simulink model "phase4_scheduler_testbed"  (R2026a)
settings: Solver=VariableStepAuto  StopTime=0.1  SampleTimeConstraint=Specified  EnableMultiTasking=on
undefined symbols (not defined in the file): D1, D3, initialControllerMeasurement, m, n, P, SupervisorTask
libraries: proctasklib x1
settings Model: Creator=The MathWorks, Inc.  LastModifiedBy=rayyu
settings SolverCC: PositivePriorityOrder=on
settings DebuggingCC: SignalInfNanChecking=error
settings HardwareCC: ProdBitPerLong=64.0  ProdLargestAtomicInteger=LongLong  ProdLargestAtomicFloat=Double  ProdHWDeviceType=ARM Compatible->ARM Cortex-A (64-bit)  HardwareBoardFeatureSet=SoCBlockset
settings RTWCC: SystemTargetFile=ert.tlc  HardwareBoard=Xilinx Zynq UltraScale+ MPSoC ZCU102 Evaluation Kit  TLCOptions="-aInlineSetEventsForThisBaseRateFcn=TLC_FALSE -aSuppressMultiTaskScheduler=TLC_FALSE  -aRateBasedStepFcn=0"  GenerateReport=on  Toolchain=Linaro AArch64 Linux v6.3.1  IncludeHyperlinkInReport=on  LaunchReport=on  GenerateTraceInfo=on  GenerateTraceReport=on  GenerateTraceReportSl=on  GenerateTraceReportSf=on  GenerateTraceReportEml=on  Description=Embedded Coder
settings ERTTargetCC: ExtModeTransport=2.0  DynamicArrayContainerType=coder::array

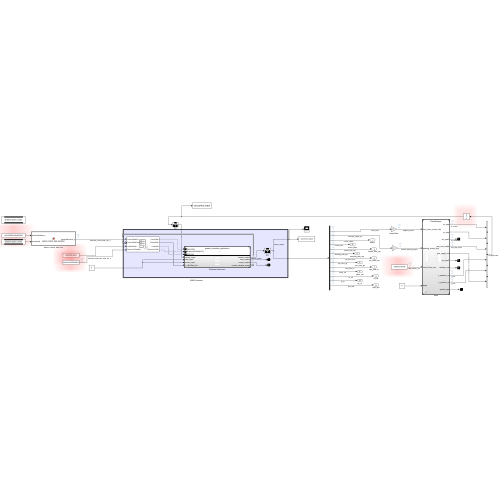
[thumbnail: Simulink's stored preview of the top-level diagram]
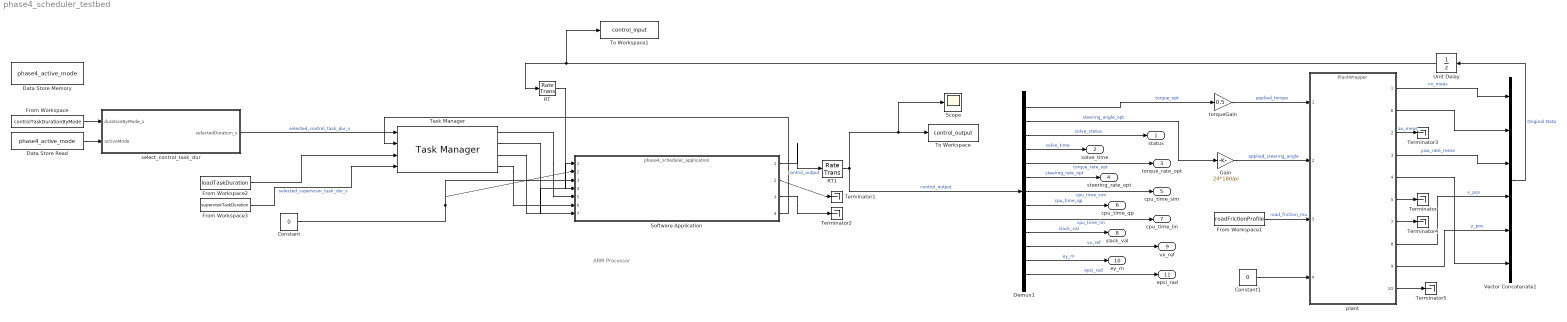
== system phase4_scheduler_testbed ==
  note: ARM Processor
  Constant : Constant  Value=0
  Constant1 : Constant  Value=0
  Data Store Memory : DataStoreMemory  DataStoreName=phase4_active_mode  WriteAfterWriteMsg=warning  InitialValue=3  ShowAdditionalParam=off  OutDataTypeStr=uint8  Dimensions=1
  Data Store Read : DataStoreRead  DataStoreName=phase4_active_mode  IndexOptions=Index vector (dialog)  Indices=1  OutputSizes=1
  Demux1 : Demux  Outputs=[1 1 1 1 1 1 1 1 1 4 1 1 1]
  From Workspace : FromWorkspace  VariableName=controlTaskDurationByMode  Interpolate=off  OutputAfterFinalValue=Holding final value
  From Workspace1 : FromWorkspace  VariableName=roadFrictionProfile  SampleTime=0.01  Interpolate=off  OutputAfterFinalValue=Holding final value
  From Workspace2 : FromWorkspace  VariableName=loadTaskDuration  Interpolate=off  OutputAfterFinalValue=Holding final value
  From Workspace3 : FromWorkspace  VariableName=supervisorTaskDuration  Interpolate=off  OutputAfterFinalValue=Holding final value
  Gain : Gain  Gain=24*180/pi
  RT : RateTransition  Deterministic=off
  RT1 : RateTransition  Deterministic=off
  Scope : Scope
      settings: ActiveDisplayYMinimum=-2.25  ActiveDisplayYMaximum=0.24999999999999994
  Software Application : ModelReference  OutputPortMessageModes=n,n,n,m  ModelNameDialog=phase4_scheduler_application.slx  SimulationMode=Normal  ScheduleRates=on  CachedPortDiscreteRates={'',0.005;'SupervisorTask',0.01;'',0.05}  ModelEventPortInfo=P:D1[0.005][0][0],P:SupervisorTask[0.01][1][0],P:D3[0.05][0][0]  HasExplicitPartitions=on  ModelReferenceVersion=14.163
  Task Manager : proctasklib/Task Manager  AllTaskData="[{\"taskName\":\"CommTask\",\"taskType\":\"Timer-driven\",\"taskEvent\":\"CommTaskEvent\",\"taskPeriod\":\"0.005\",\"taskPriority\":\"50\",\"coreSelection\":\"Specified core\",\"coreNum\":\"0\",\"dropOverranTasks\":false,\"playbackRecorded\":false,\"diagnosticsFile\":\"\",\"taskDurationSource\":\"Dialog\",\"taskDuration\":1E-6,\"taskDurationDeviation\":0,\"logExecutionData\":true,\"logDroppedTasks\":false,\"version\":\"2.6\",\"taskDurationData\":{\"percent\":\"100\",\"mean\":\"0.0005\",\"dev\":\"0\",\"min\":\"0.0005\",\"max\":\"0.0005\"},\"taskEventSource\":\"Internal\",\"taskEventSourceAssignmentType\":\"AutoAssigned\",\"taskEventSourceType\":\"Unspecified\",\"taskEventGroup\":\"Unspecified\",\"taskEventInterrupt\":\"Unspecified\",\"taskEventOrder\":1,\"taskDisablePremption\":false,\"taskClearInterruptFlagsAtEndOfEvent\":false},{\"taskName\":\"ControlTask\",\"taskType\":\"Event-driven\",\"taskEvent\":\"ControlTaskEvent\",\"taskPeriod\":\"0.01\",\"taskPriority\":\"50\",\"coreSelection\":\"Specified core\",\"coreNum\":\"0\",\"dropOverranTasks\":false,\"playbackRecorded\":false,\"diagnosticsFile\":\"\",\"taskDurationSource\":\"Input port\",\"taskDuration\":1E-6,\"taskDurationDeviation\":0,\"logExecutionData\":true,\"logDroppedTasks\":false,\"version\":\"2.6\",\"taskDurationData\":{\"percent\":\"100\",\"mean\":\"1e-06\",\"dev\":\"0\",\"min\":\"1e-06\",\"max\":\"1e-06\"},\"taskEventSource\":\"Unspecified\",\"taskEventSourceAssignmentType\":\"Unassigned\",\"taskEventSourceType\":\"Unspecified\",\"taskEventGroup\":\"Unspecified\",\"taskEventInterrupt\":\"Unspecified\",\"taskEventOrder\":1,\"taskDisablePremption\":false,\"taskClearInterruptFlagsAtEndOfEvent\":false},{\"taskName\":\"LoadTask\",\"taskType\":\"Timer-driven\",\"taskEvent\":\"newTask1Event\",\"taskPeriod\":\"0.05\",\"taskPriority\":\"50\",\"coreSelection\":\"Specified core\",\"coreNum\":\"0\",\"dropOverranTasks\":false,\"playbackRecorded\":false,\"diagnosticsFile\":\"\",\"taskDurationSource\":\"Input port\",\"taskDuration\":1E-6,\"taskDurationDeviation\":0,\"logExecutionData\":true,\"logDroppedTasks\":false,\"version\":\"2.6\",\"taskDurationData\":{\"percent\":\"100\",\"mean\":\"1e-06\",\"dev\":\"0\",\"min\":\"1e-06\",\"max\":\"1e-06\"},\"taskEventSource\":\"Internal\",\"taskEventSourceAssignmentType\":\"AutoAssigned\",\"taskEventSourceType\":\"Unspecified\",\"taskEventGroup\":\"Unspecified\",\"taskEventInterrupt\":\"Unspecified\",\"taskEventOrder\":1,\"taskDisablePremption\":false,\"taskClearInterruptFlagsAtEndOfEvent\":false},{\"taskName\":\"SupervisorTask\",\"taskType\":\"Timer-driven\",\"taskEvent\":\"SchedulerTaskEvent\",\"taskPeriod\":\"0.01\",\"taskPriority\":\"51\",\"coreSelection\":\"Specified core\",\"coreNum\":\"0\",\"dropOverranTasks\":false,\"playbackRecorded\":false,\"diagnosticsFile\":\"\",\"taskDurationSource\":\"Input port\",\"taskDuration\":1E-6,\"taskDurationDeviation\":0,\"logExecutionData\":true,\"logDroppedTasks\":false,\"version\":\"2.6\",\"taskDurationData\":{\"percent\":\"100\",\"mean\":\"0.00005\",\"dev\":\"0\",\"min\":\"0.00005\",\"max\":\"0.00005\"},\"taskEventSource\":\"Internal\",\"taskEventSourceAssignmentType\":\"AutoAssigned\",\"taskEventSourceType\":\"Unspecified\",\"taskEventGroup\":\"Unspecified\",\"taskEventInterrupt\":\"Unspecified\",\"taskEventOrder\":1,\"taskDisablePremption\":false,\"taskClearInterruptFlagsAtEndOfEvent\":false}]"  EnableTaskSimulation=on  StreamToSDI=on  WriteToFile=off  OverwriteFile=off  SupportEventPorts=on  UseScheduleEditor=off  CustomizationInfo=''
  Terminator{,1..5} (6 alike) : Terminator
  To Workspace : ToWorkspace  VariableName=control_output  SaveFormat=Timeseries  SampleTime=-1
  To Workspace1 : ToWorkspace  VariableName=control_input  SaveFormat=Timeseries  SampleTime=-1
  Unit Delay : UnitDelay  InitialCondition=initialControllerMeasurement  SampleTime=-1
  Vector Concatenate1 : Concatenate  NumInputs=6
  plant : ModelReference  ModelNameDialog=PlantWrapper.slx  SimulationMode=Normal  ModelReferenceVersion=1.23
      settings: PortSchema="{\"entries\":[{\"content\":{\"sides\":[{\"content\":{\"connectorIds\":[\"In1\",\"In2\",\"In3\",\"In4\"]},\"type\":\"ConnectorPlacement.EquallySpacedRectSide\",\"uuid\":\"bf665537-3fd8-4fa0-88a8-2cb308153754\"},{\"content\":{\"connectorIds\":[\"Out1\",\"Out6\",\"Out2\",\"Out3\",\"Out4\",\"Out5\",\"Out7\",\"Out8\",\"Out9\",\"Out10\"],\"side\":\"RIGHT\"},\"type\":\"ConnectorPlacement.EquallySpacedRectSide\",\"uuid\":\"a274990e-adc2-49b8-8679-a2f39e53ce6e\"},{\"content\":{\"side\":\"TOP\"},\"type\":\"ConnectorPlacement.EquallySpacedRectSide\",\"uuid\":\"963f9bff-e020-46b1-9958-cad0758083aa\"}]},\"type\":\"ConnectorPlacement.EquallySpacedConnector\",\"uuid\":\"fb8d0fca-1617-49ee-84dd-83e8b757a297\"}],\"packageUris\":[\"http://schema.mathworks.com/mf0/Connector/R2020b\"],\"version\":\"1.0\"}"
  select_control_task_dur : MATLAB Function  TreatAsAtomicUnit=on
  torqueGain : Gain  Gain=0.5
  status : Outport
  solve_time : Outport  Port=2
  torque_rate_opt : Outport  Port=3
  steering_rate_opt : Outport  Port=4
  cpu_time_sim : Outport  Port=5
  cpu_time_qp : Outport  Port=6
  cpu_time_lin : Outport  Port=7
  slack_val : Outport  Port=8
  vx_ref : Outport  Port=9
  ey_m : Outport  Port=10
  epsi_rad : Outport  Port=11
  wires:
  RT1/1 -> Scope/1, To Workspace/1, Demux1/1  "control_output"
  Vector Concatenate1/1 -> Unit Delay/1  "Original Data"
  Software Application/2 -> Terminator1/1
  Constant/1 -> Software Application/2, Software Application/3
  Task Manager/1 -> Software Application/5
  select_control_task_dur/1(selectedDuration_s) -> Task Manager/1  "selected_control_task_dur_s"
  Demux1/1 -> torqueGain/1  "torque_opt"
  Demux1/2 -> Gain/1  "steering_angle_opt"
  plant/1 -> Vector Concatenate1/1  "vx_meas"
  plant/6 -> Vector Concatenate1/2
  plant/3 -> Vector Concatenate1/3  "yaw_rate_meas"
  plant/8 -> Vector Concatenate1/4  "x_pos"
  plant/9 -> Vector Concatenate1/5  "y_pos"
  plant/4 -> Vector Concatenate1/6
  plant/2 -> Terminator3/1  "ax_meas"
  plant/5 -> Terminator/1
  plant/7 -> Terminator4/1
  torqueGain/1 -> plant/1  "applied_torque"
  Gain/1 -> plant/2  "applied_steering_angle"
  Constant1/1 -> plant/4
  From Workspace1/1 -> plant/3  "road_friction_mu"
  plant/10 -> Terminator5/1
  Unit Delay/1 -> RT/1, To Workspace1/1
  From Workspace2/1 -> Task Manager/3
  Task Manager/2 -> Software Application/4
  Task Manager/3 -> Software Application/7
  Software Application/3 -> Terminator2/1
  Software Application/4 -> Task Manager/2
  Task Manager/4 -> Software Application/6
  RT/1 -> Software Application/1
  Software Application/1 -> RT1/1  "control_output"
  Demux1/6 -> steering_rate_opt/1  "steering_rate_opt"
  Demux1/4 -> solve_time/1  "solve_time"
  Demux1/7 -> cpu_time_sim/1  "cpu_time_sim"
  Demux1/9 -> cpu_time_lin/1  "cpu_time_lin"
  Demux1/8 -> cpu_time_qp/1  "cpu_time_qp"
  Demux1/10 -> slack_val/1  "slack_val"
  Demux1/5 -> torque_rate_opt/1  "torque_rate_opt"
  Demux1/3 -> status/1  "solve_status"
  Demux1/11 -> vx_ref/1  "vx_ref"
  Demux1/12 -> ey_m/1  "ey_m"
  Demux1/13 -> epsi_rad/1  "epsi_rad"
  From Workspace3/1 -> Task Manager/4  "selected_supervisor_task_dur_s"
  From Workspace/1 -> select_control_task_dur/1(durationByMode_s)
  Data Store Read/1 -> select_control_task_dur/2(activeMode)

== matlab function phase4_scheduler_testbed/select_control_task_dur ==
  data: durationByMode_s input double; selectedDuration_s output double; activeMode input
function selectedDuration_s = ...
    select_control_task_duration( ...
        durationByMode_s, activeMode)

modeIndex = round(double(activeMode));
modeIndex = min(max(modeIndex, 1), 3);

selectedDuration_s = ...
    durationByMode_s(modeIndex);

end
